simulink model "Assignment"  (R2020b)
settings: Solver=VariableStepAuto  StartTime=0.0  StopTime=2628000  RelTol=1e-3
libraries: ET3036TU_model_library_2020a_fix x8, powerlib_meascontrol x2, powerlib x1
settings Model: SimulationMode=accelerator  Creator=lpantea  LastModifiedBy=cparengkuan

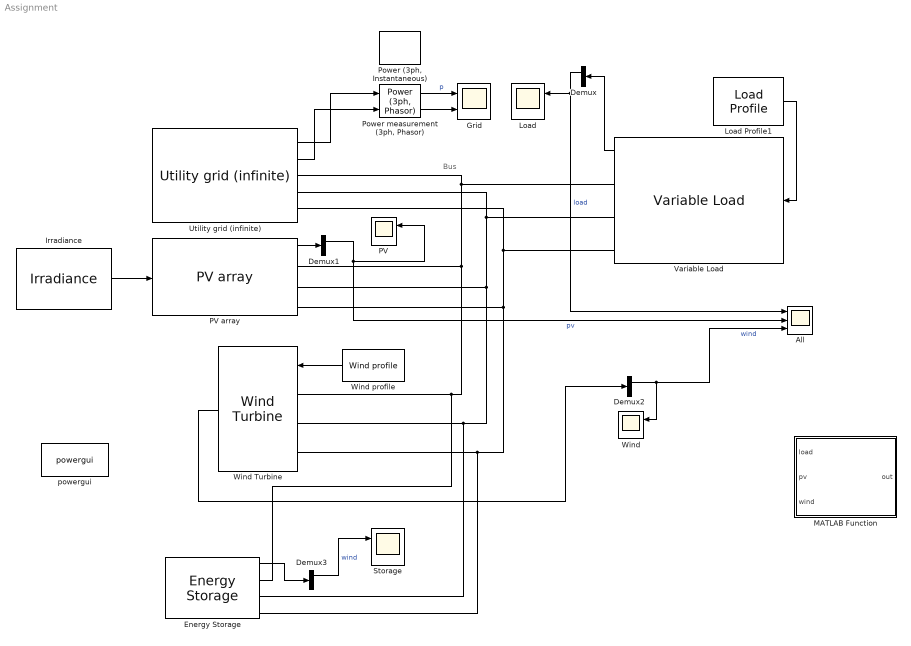
== system Assignment ==
  note: Bus
  All : Scope  NumInputPorts=3
  Demux{,1..3} (4 alike) : Demux  Outputs=2
  Energy Storage : ET3036TU_model_library_2020a_fix/Energy Storage  Vn=230*sqrt(3)  Fn=50  PnomkW=100  kWh_Rated=500  Efficiency=96  LimitVec=[100 0]  RechargeSOC=50  Precharge=100  autoRecharge=off  Initial_kWh_pc=50  PQvec=[0 0]
  Grid : Scope  NumInputPorts=2
  Irradiance : ET3036TU_model_library_2020a_fix/Irradiance
  Load : Scope  NumInputPorts=2
  Load Profile1 : ET3036TU_model_library_2020a_fix/Load Profile
  MATLAB Function : MATLAB Function  AncestorBlock=ET3036TU_model_library_2020a_fix/MATLAB Function  TreatAsAtomicUnit=on
  PV : Scope  NumInputPorts=2
  "PV array " : ET3036TU_model_library_2020a_fix/PV array   Efficiency=0.2  Area=100  Vnom=230*sqrt(3)  fnom=50
  "Power (3ph, Instantaneous)" : powerlib_meascontrol/Measurements/Power (3ph, Instantaneous)
  "Power measurement (3ph, Phasor)" : powerlib_meascontrol/Measurements/Power (3ph, Phasor)
      settings: SourceProductBaseCode=PS
  Storage : Scope  NumInputPorts=2
  Utility grid (infinite) : ET3036TU_model_library_2020a_fix/Utility grid (infinite)  Vgrid=230*sqrt(3)  fnom=50
  Variable Load : ET3036TU_model_library_2020a_fix/Variable Load  Vn=230*sqrt(3)  Fn=50  PF=1  Load0=0
  Wind : Scope  NumInputPorts=2
  "Wind Turbine " : ET3036TU_model_library_2020a_fix/Wind Turbine     Unom=15  Umax=25  Umin=5  Pselect=1: Simple Cubic Power  fnom=50  Vnom=230*sqrt(3)  Pnom=20  rp=5  Cp=16/27  rho=1.225  Uvec=[1:1:30]  Pvec=[0,0,0,0,21359.3750000000,58193.5000000000,104316.125000000,157104.500000000,213935.875000000,272187.500000000,329236.625000000,382460.500000000,429236.375000000,466941.500000000,492953.125000000,500000,500000,500000,500000,500000,500000,500000,500000,500000,500000,0,0,0,0,0]  Tp=0.1  Tq=1  ReactP=0
  Wind profile : ET3036TU_model_library_2020a_fix/Wind profile
  powergui : powerlib/powergui  Priority=1  SimulationMode=Phasor  SampleTime=50e-4  frequency=50  Iterations=50  frequencyindice=50  Pbase=100e6  ErrMax=1e-4  UnitsV=kV  UnitsW=MW  buscounter=0  FunctionMessages=off  echomessages=off  EnableUseOfTLC=off  CurrentSourceSwitches=off  DisableSnubberDevices=off  DisableRonSwitches=off  DisableVfSwitches=off  DisplayEquations=off  AutomaticDiscreteSolvers=off  SolverType=Tustin/Backward Euler (TBE)  Interpol=off  ExternalGateDelay=off  methode=off  Ts=100  x0status=blocks  SPID=on  SwTol=0  HookPort=off  NonlinearTolerance=1e-4  nMaxIteration=100  ContinueOnMaxIteration=off  RestoreLinks=warning  ResistiveCurrentMeasurement=off  Frange=[0:2:500]  Ylog=off  Xlog=on  ShowGrid=off  save=off  variable=ZData  structure=0  ZoomFFT=off  StartTime=0.0  cycles=1  DisplayStyle=1  fundamental=60  FreqAxis=off  MaxFrequency=1000  frequencyindicesteady=1  RmsSteady=1  display=off
  wires:
  Load Profile1/1 -> Variable Load/1
  Wind profile/1 -> "Wind Turbine "/1
  Irradiance/1 -> "PV array "/1
  Variable Load/1 -> Demux/1
  Demux/1 -> Load/1, All/1  "load"
  "PV array "/1 -> Demux1/1
  Demux1/1 -> PV/1, All/2  "pv"
  "Wind Turbine "/1 -> Demux2/1
  Demux2/1 -> Wind/1, All/3  "wind"
  Utility grid (infinite)/1 -> "Power measurement (3ph, Phasor)"/1
  Utility grid (infinite)/2 -> "Power measurement (3ph, Phasor)"/2
  "Power measurement (3ph, Phasor)"/1 -> Grid/1  "p"
  "Power measurement (3ph, Phasor)"/2 -> Grid/2
  Energy Storage/1 -> Demux3/1
  Demux3/1 -> Storage/1  "wind"
  connections:
  Variable Load/RConn3 -- Utility grid (infinite)/RConn3 -- "PV array "/RConn3 -- Energy Storage/RConn3 -- "Wind Turbine "/LConn3
  Variable Load/RConn2 -- Utility grid (infinite)/RConn2 -- "PV array "/RConn2 -- Energy Storage/RConn2 -- "Wind Turbine "/LConn2
  Utility grid (infinite)/RConn1 -- "PV array "/RConn1 -- Energy Storage/RConn1 -- "Wind Turbine "/LConn1 -- Variable Load/RConn1

== matlab function Assignment/MATLAB Function ==
  data: load input; out output; pv input; wind input
function out = Controller(load, pv, wind)
    return (pv + wind - load;
    % load - the load demand (W)
    % pv   - the solar generated power (W)
    % wind - the wind generated power (W)
    % negative if discharge, positive otherwise
end
